simulink model "torque_control_model_3"  (R2017b)
settings: Solver=FixedStepAuto  StartTime=0.0  StopTime=.1  FixedStep=1e-6  RelTol=1e-3
InitFcn:
  | BLDC_motor_constants_2;
  | clc;
  | 
  | f=5000;           % Reference frequency
  | fs=4000;      % Switching frequency
  | m=1;           % Modulation index
  | 
  | Ts=10e-6;    % Sampling time of devices
values from neighbouring files (symbols this model uses):
  A = [-terminal_resistance/terminal_inductance, 0, 0 ... (first row only)    [BLDC_motor_constants_2.m]    (also in forward_dynamics.m = pinv(Z) * V; inverse_dynamics.m = -pinv(Z) * v)
  B = [2/(3 * terminal_inductance), 1/(3 * terminal_inductance), 0 ... (first row only)    [BLDC_motor_constants_2.m]    (also in forward_dynamics.m = pinv(Z)/gear_ratio)
  C = [1, 0, 0 ... (first row only)    [BLDC_motor_constants_2.m]
  kf = 0.001    [BLDC_motor_constants_2.m]
  pole_pairs = 8    [BLDC_motor_constants_2.m]
  rotor_inertia = 0.000181    [BLDC_motor_constants_2.m]
  speed_constant = 259    [BLDC_motor_constants_2.m]
  torque_constant = 36.9    [BLDC_motor_constants_2.m]
libraries: simulink x3
settings Model: Creator=Zach  LastModifiedBy=Zach

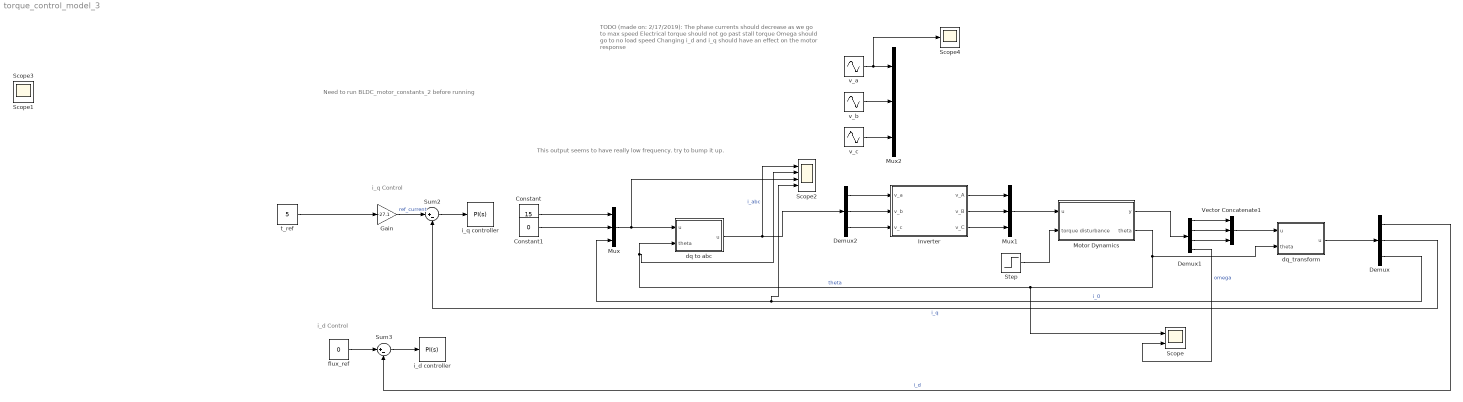
== system torque_control_model_3 ==
  note: TODO (made on: 2/17/2019):
      | The phase currents should decrease as we go to max speed
      | Electrical torque should not go past stall torque
      | Omega should go to no load speed
      | Changing i_d and i_q should have an effect on the motor response
  note: This output seems to have really low frequency. try to bump it up.
  note: i_d Control
  note: i_q Control
  note: Need to run BLDC_motor_constants_2 before running
  Constant : Constant  Value=15
  Constant1 : Constant  Value=0
  Demux : Demux  Outputs=3
  Demux1 : Demux
  Demux2 : Demux  Outputs=3
  Gain : Gain  Gain=-27.1
  Inverter : Subsystem
  Motor Dynamics : Subsystem
  Mux : Mux  Inputs=3
  Mux1 : Mux  Inputs=3
  Mux2 : Mux  Inputs=3
  Scope : Scope  NumInputPorts=2
  Scope2 : Scope  NumInputPorts=4
  Scope4 : Scope
  Step : Step  After=-.25  SampleTime=0
  Sum2 : Sum  Inputs=|+-
  Sum3 : Sum  Inputs=|+-
  Vector Concatenate1 : Concatenate  NumInputs=3
  dq to abc : MATLAB Function  TreatAsAtomicUnit=on
  dq_transform : MATLAB Function  TreatAsAtomicUnit=on
  flux_ref : Constant  Value=0
  i_d controller : simulink/Continuous/PID Controller  Controller=PI  TimeDomain=Continuous-time  SampleTime=-1  IntegratorMethod=Forward Euler  FilterMethod=Forward Euler  Form=Parallel  UseFilter=on  ControllerParametersSource=internal  P=20  I=1  D=0  N=100  InitialConditionSource=internal  InitialConditionForIntegrator=0  InitialConditionForFilter=0  ExternalReset=none  LimitOutput=off  UpperSaturationLimit=inf  LowerSaturationLimit=-inf  LinearizeAsGain=on  AntiWindupMode=none  Kb=1  TrackingMode=off  Kt=1  PParamMin=[]  PParamMax=[]  IParamMin=[]  IParamMax=[]  DParamMin=[]  DParamMax=[]  NParamMin=[]  NParamMax=[]  KbParamMin=[]  KbParamMax=[]  KtParamMin=[]  KtParamMax=[]  POutMin=[]  POutMax=[]  IOutMin=[]  IOutMax=[]  DOutMin=[]  DOutMax=[]  NOutMin=[]  NOutMax=[]  KbOutMin=[]  KbOutMax=[]  KtOutMin=[]  KtOutMax=[]  IntegratorOutMin=[]  IntegratorOutMax=[]  FilterOutMin=[]  FilterOutMax=[]  SumOutMin=[]  SumOutMax=[]  SumI1OutMin=[]  SumI1OutMax=[]  SumI2OutMin=[]  SumI2OutMax=[]  SumI3OutMin=[]  SumI3OutMax=[]  SumDOutMin=[]  SumDOutMax=[]  SaturationOutMin=[]  SaturationOutMax=[]  IntegratorContinuousStateAttributes=''  IntegratorStateMustResolveToSignalObject=off  IntegratorRTWStateStorageClass=Auto  FilterContinuousStateAttributes=''  FilterStateMustResolveToSignalObject=off  FilterRTWStateStorageClass=Auto  DifferentiatorICPrevScaledInput=0  DifferentiatorOutMin=[]  DifferentiatorOutMax=[]  InitialConditionSetting=State (most efficient)  FilterDiffOutCoefMin=[]  FilterDiffOutCoefMax=[]  SumDenOutMin=[]  SumDenOutMax=[]  SumNumOutMin=[]  SumNumOutMax=[]  ReciprocalOutMin=[]  ReciprocalOutMax=[]  DivideOutMin=[]  DivideOutMax=[]  TunerSelectOption=Transfer Function Based (PID Tuner App)
  i_q controller : simulink/Continuous/PID Controller  Controller=PI  TimeDomain=Continuous-time  SampleTime=-1  IntegratorMethod=Forward Euler  FilterMethod=Forward Euler  Form=Parallel  UseFilter=on  ControllerParametersSource=internal  P=1  I=1  D=0  N=100  InitialConditionSource=internal  InitialConditionForIntegrator=0  InitialConditionForFilter=0  ExternalReset=none  LimitOutput=off  UpperSaturationLimit=inf  LowerSaturationLimit=-inf  LinearizeAsGain=on  AntiWindupMode=none  Kb=1  TrackingMode=off  Kt=1  PParamMin=[]  PParamMax=[]  IParamMin=[]  IParamMax=[]  DParamMin=[]  DParamMax=[]  NParamMin=[]  NParamMax=[]  KbParamMin=[]  KbParamMax=[]  KtParamMin=[]  KtParamMax=[]  POutMin=[]  POutMax=[]  IOutMin=[]  IOutMax=[]  DOutMin=[]  DOutMax=[]  NOutMin=[]  NOutMax=[]  KbOutMin=[]  KbOutMax=[]  KtOutMin=[]  KtOutMax=[]  IntegratorOutMin=[]  IntegratorOutMax=[]  FilterOutMin=[]  FilterOutMax=[]  SumOutMin=[]  SumOutMax=[]  SumI1OutMin=[]  SumI1OutMax=[]  SumI2OutMin=[]  SumI2OutMax=[]  SumI3OutMin=[]  SumI3OutMax=[]  SumDOutMin=[]  SumDOutMax=[]  SaturationOutMin=[]  SaturationOutMax=[]  IntegratorContinuousStateAttributes=''  IntegratorStateMustResolveToSignalObject=off  IntegratorRTWStateStorageClass=Auto  FilterContinuousStateAttributes=''  FilterStateMustResolveToSignalObject=off  FilterRTWStateStorageClass=Auto  DifferentiatorICPrevScaledInput=0  DifferentiatorOutMin=[]  DifferentiatorOutMax=[]  InitialConditionSetting=State (most efficient)  FilterDiffOutCoefMin=[]  FilterDiffOutCoefMax=[]  SumDenOutMin=[]  SumDenOutMax=[]  SumNumOutMin=[]  SumNumOutMax=[]  ReciprocalOutMin=[]  ReciprocalOutMax=[]  DivideOutMin=[]  DivideOutMax=[]  TunerSelectOption=Transfer Function Based (PID Tuner App)
  t_ref : Constant  Value=5
  v_a : Sin  Frequency=pi*2*f  Phase=pi/2  SampleTime=0
  v_b : Sin  Frequency=f*2*pi  Phase=pi/2 -2*pi/3  SampleTime=0
  v_c : Sin  Frequency=12  Phase=pi/2+2*pi/3  SampleTime=0
  Scope1 : Scope
  Scope3 : Scope
  wires:
  Gain/1 -> Sum2/1  "ref_current"
  Sum2/1 -> i_q controller/1
  Demux/2 -> Sum2/2  "i_q"
  flux_ref/1 -> Sum3/1
  Sum3/1 -> i_d controller/1
  Demux/1 -> Sum3/2  "i_d"
  Demux/3 -> Scope2/4, Mux/3  "i_0"
  Step/1 -> Motor Dynamics/2(torque disturbance)
  Motor Dynamics/1(y) -> Demux1/1
  Demux1/2 -> Vector Concatenate1/2
  Demux1/1 -> Vector Concatenate1/1
  Demux1/3 -> Vector Concatenate1/3
  Motor Dynamics/2(theta) -> dq_transform/2(theta), Scope2/2, dq to abc/2(theta), Scope/1  "theta"
  Vector Concatenate1/1 -> dq_transform/1("u ")
  dq_transform/1(u) -> Demux/1
  Demux1/4 -> Scope/2  "omega"
  Constant/1 -> Mux/1
  Constant1/1 -> Mux/2
  t_ref/1 -> Gain/1
  Mux/1 -> Scope2/3, dq to abc/1("u ")
  Demux2/1 -> Inverter/1(v_a)
  Demux2/2 -> Inverter/2(v_b)
  Demux2/3 -> Inverter/3(v_c)
  Inverter/2(v_B) -> Mux1/2
  Inverter/1(v_A) -> Mux1/1
  Inverter/3(v_C) -> Mux1/3
  Mux1/1 -> Motor Dynamics/1(u)
  v_b/1 -> Mux2/2
  v_a/1 -> Scope4/1, Mux2/1
  v_c/1 -> Mux2/3
  dq to abc/1(u) -> Demux2/1, Scope2/1  "i_abc"

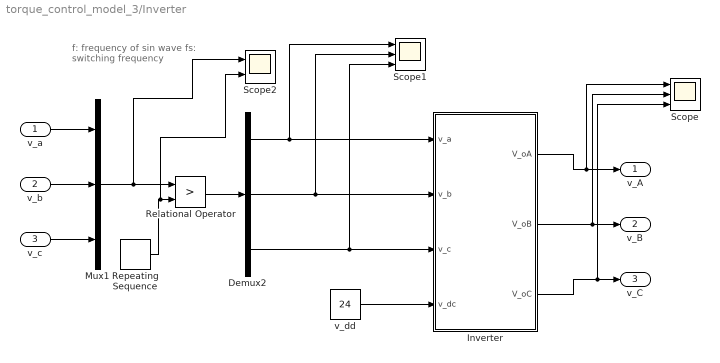
== system torque_control_model_3/Inverter ==
  note: f: frequency of sin wave
      | fs: switching frequency
  v_a : Inport
  v_b : Inport  Port=2
  v_c : Inport  Port=3
  Demux2 : Demux  Outputs=3
  Inverter : Subsystem
  Mux1 : Mux  Inputs=3
  Relational Operator : RelationalOperator  Operator=>  OutDataTypeStr=boolean  RndMeth=Simplest
  Repeating Sequence : simulink/Sources/Repeating Sequence  rep_seq_t=[0 0.25/fs 0.5/fs 0.75/fs 1/fs]  rep_seq_y=[1 0 -1 0 1]
  Scope : Scope  NumInputPorts=3
  Scope1 : Scope  NumInputPorts=3
  Scope2 : Scope  NumInputPorts=2
  v_dd : Constant  Value=24
  v_A : Outport
  v_B : Outport  Port=2
  v_C : Outport  Port=3
  wires:
  Relational Operator/1 -> Demux2/1
  Inverter/1(V_oA) -> Scope/1, v_A/1
  v_c/1 -> Mux1/3
  v_a/1 -> Mux1/1
  Demux2/3 -> Scope1/3, Inverter/3(v_c)
  Repeating Sequence/1 -> Scope2/2, Relational Operator/2
  v_b/1 -> Mux1/2
  Inverter/3(V_oC) -> Scope/3, v_C/1
  Demux2/1 -> Scope1/1, Inverter/1(v_a)
  Mux1/1 -> Scope2/1, Relational Operator/1
  v_dd/1 -> Inverter/4(v_dc)
  Demux2/2 -> Scope1/2, Inverter/2(v_b)
  Inverter/2(V_oB) -> Scope/2, v_B/1

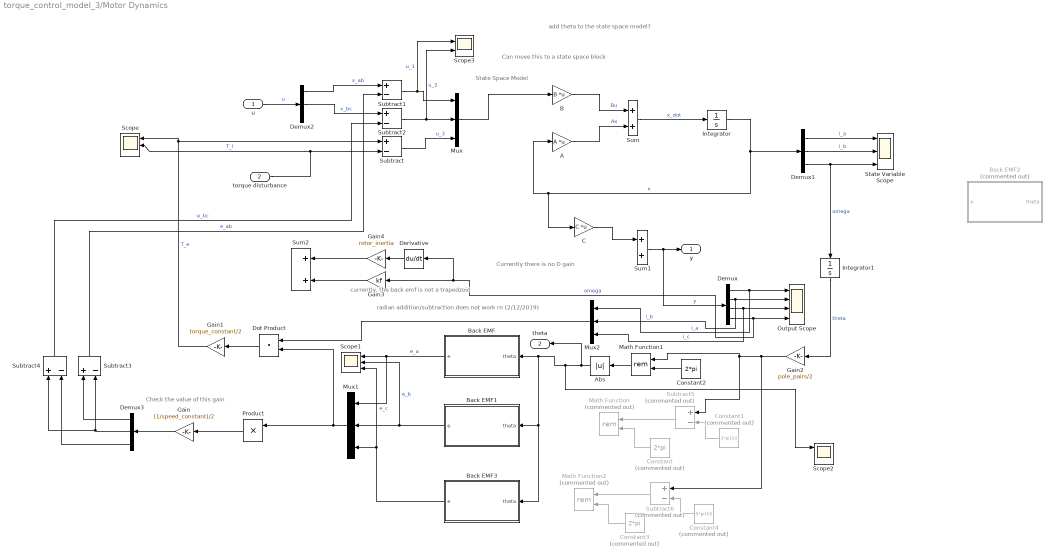
== system torque_control_model_3/Motor Dynamics ==
  note: radian addition/subtraction does not work rn (2/12/2019)
  note: add theta to the state space model?
  note: Check the value of this gain
  note: Can move this to a state space block
  note: currently, the back emf is not a trapedzoid
  note: Currently there is no D gain
  note: State Space Model
  u : Inport
  torque disturbance : Inport  Port=2
  A : Gain  Gain=A  Multiplication=Matrix(K*u)
  Abs : Abs
  B : Gain  Gain=B  Multiplication=Matrix(K*u)
  Back EMF : Subsystem
  Back EMF1 : Subsystem
  Back EMF2 : Subsystem  Commented=on
  Back EMF3 : Subsystem
  C : Gain  Gain=C  Multiplication=Matrix(K*u)
  Constant : Constant  Commented=on  Value=2*pi
  Constant1 : Constant  Commented=on  Value=2*pi()/3
  Constant2 : Constant  Value=2*pi
  Constant3 : Constant  Commented=on  Value=2*pi
  Constant4 : Constant  Commented=on  Value=5*pi()/3
  Demux : Demux
  Demux1 : Demux  Outputs=3
  Demux2 : Demux  Outputs=3
  Demux3 : Demux  Outputs=3
  Derivative : Derivative
  Dot Product : DotProduct  InputSameDT=on  OutDataTypeStr=Inherit: Inherit via internal rule
  Gain : Gain  Gain=(1/speed_constant)/2
  Gain1 : Gain  Gain=torque_constant/2
  Gain2 : Gain  Gain=pole_pairs/2
  Gain3 : Gain  Gain=kf
  Gain4 : Gain  Gain=rotor_inertia
  Integrator : Integrator
  Integrator1 : Integrator
  Math Function : Math  Commented=on  Operator=rem  SaturateOnIntegerOverflow=on
  Math Function1 : Math  Operator=rem  SaturateOnIntegerOverflow=on
  Math Function2 : Math  Commented=on  Operator=rem  SaturateOnIntegerOverflow=on
  Mux : Mux  Inputs=3
  Mux1 : Mux  Inputs=3
  Mux2 : Mux  Inputs=3
  Output Scope : Scope  NumInputPorts=4
  Product : Product
  Scope : Scope  NumInputPorts=3
  Scope1 : Scope  NumInputPorts=3
  Scope2 : Scope  NumInputPorts=3
  Scope3 : Scope  NumInputPorts=2
  State Variable Scope : Scope  NumInputPorts=3
  Subtract{,1..4} (5 alike) : Sum  Inputs=+-
  Subtract5 : Sum  Commented=on  Inputs=+-
  Subtract6 : Sum  Commented=on  Inputs=+-
  Sum : Sum
  Sum1 : Sum
  Sum2 : Sum
  y : Outport
  theta : Outport  Port=2
  wires:
  B/1 -> Sum/1  "Bu"
  A/1 -> Sum/2  "Ax"
  Sum/1 -> Integrator/1  "x_dot"
  Integrator/1 -> Demux1/1, C/1, A/1  "x"
  C/1 -> Sum1/1
  Sum1/1 -> Demux/1, y/1  "y"
  Demux/1 -> Mux2/1, Output Scope/1  "i_a"
  Demux/2 -> Mux2/2, Output Scope/2  "i_b"
  Demux/3 -> Mux2/3, Output Scope/3  "i_c"
  Demux/4 -> Derivative/1, Gain3/1, Output Scope/4  "omega"
  Demux1/1 -> State Variable Scope/1  "i_a"
  Demux1/2 -> State Variable Scope/2  "i_b"
  Demux1/3 -> State Variable Scope/3, Integrator1/1  "omega"
  Mux/1 -> B/1
  u/1 -> Demux2/1  "u"
  torque disturbance/1 -> Scope/2, Subtract/2  "T_l"
  Demux2/1 -> Subtract1/1  "v_ab"
  Demux2/2 -> Subtract2/1  "v_bc"
  Subtract2/1 -> Scope3/2, Mux/2  "u_2"
  Subtract1/1 -> Scope3/1, Mux/1  "u_1"
  Subtract/1 -> Mux/3  "u_3"
  Subtract3/1 -> Subtract1/2  "e_ab"
  Subtract4/1 -> Subtract2/2  "e_bc"
  Mux1/1 -> Dot Product/2, Product/1
  Product/1 -> Gain/1
  Gain/1 -> Demux3/1
  Demux3/1 -> Subtract3/1
  Demux3/2 -> Subtract4/1, Subtract3/2
  Demux3/3 -> Subtract4/2
  Mux2/1 -> Dot Product/1
  Dot Product/1 -> Gain1/1
  Gain1/1 -> Scope/1, Subtract/1  "T_e"
  Integrator1/1 -> Gain2/1  "theta"
  Constant/1 -> Math Function/2
  Constant1/1 -> Subtract5/2
  Subtract5/1 -> Math Function/1
  Constant2/1 -> Math Function1/2
  Constant4/1 -> Subtract6/2
  Constant3/1 -> Math Function2/2
  Subtract6/1 -> Math Function2/1
  Gain2/1 -> Subtract6/1, Subtract5/1, Math Function1/1
  Back EMF/1(e) -> Mux1/1, Scope1/1  "e_a"
  Back EMF1/1(e) -> Scope1/2, Mux1/2  "e_b"
  Back EMF3/1(e) -> Scope1/3, Mux1/3  "e_c"
  Derivative/1 -> Gain4/1
  Gain3/1 -> Sum2/2
  Gain4/1 -> Sum2/1
  Math Function1/1 -> Abs/1
  Abs/1 -> theta/1, Scope2/1, Back EMF3/1(theta), Back EMF1/1(theta), Back EMF/1(theta)

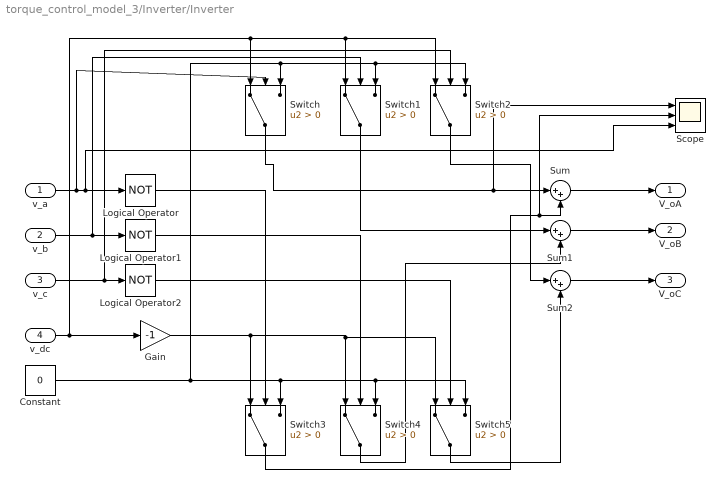
== system torque_control_model_3/Inverter/Inverter ==
  v_a : Inport
  v_b : Inport  Port=2
  v_c : Inport  Port=3
  v_dc : Inport  Port=4
  Constant : Constant  Value=0
  Gain : Gain  Gain=-1
  Logical Operator : Logic  Operator=NOT  AllPortsSameDT=off  OutDataTypeStr=boolean
  Logical Operator1 : Logic  Operator=NOT  AllPortsSameDT=off  OutDataTypeStr=boolean
  Logical Operator2 : Logic  Operator=NOT  AllPortsSameDT=off  OutDataTypeStr=boolean
  Scope : Scope  NumInputPorts=3
  Sum : Sum  Inputs=|++
  Sum1 : Sum  Inputs=|++
  Sum2 : Sum  Inputs=|++
  Switch{,1..5} (6 alike) : Switch  Criteria=u2 > Threshold
  V_oA : Outport
  V_oB : Outport  Port=2
  V_oC : Outport  Port=3
  wires:
  v_a/1 -> Switch/2, Scope/3, Logical Operator/1
  v_b/1 -> Switch1/2, Logical Operator1/1
  v_c/1 -> Switch2/2, Logical Operator2/1
  Logical Operator/1 -> Switch3/2
  Logical Operator1/1 -> Switch4/2
  Logical Operator2/1 -> Switch5/2
  v_dc/1 -> Switch2/1, Switch1/1, Switch/1, Gain/1
  Gain/1 -> Switch5/1, Switch4/1, Switch3/1
  Constant/1 -> Switch2/3, Switch1/3, Switch/3, Switch5/3, Switch4/3, Switch3/3
  Sum/1 -> V_oA/1
  Sum1/1 -> V_oB/1
  Sum2/1 -> V_oC/1
  Switch/1 -> Sum/1, Scope/1
  Switch3/1 -> Scope/2, Sum/2
  Switch1/1 -> Sum1/1
  Switch4/1 -> Sum1/2
  Switch2/1 -> Sum2/1
  Switch5/1 -> Sum2/2

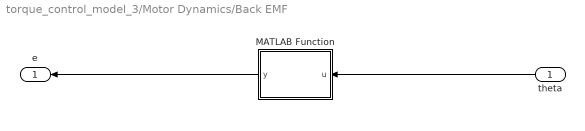
== system torque_control_model_3/Motor Dynamics/Back EMF ==
  theta : Inport
  MATLAB Function : MATLAB Function  TreatAsAtomicUnit=on
  e : Outport
  wires:
  theta/1 -> MATLAB Function/1(u)
  MATLAB Function/1(y) -> e/1

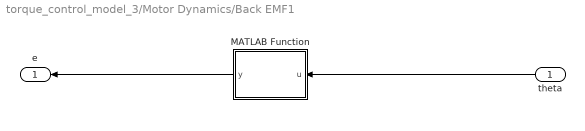
== system torque_control_model_3/Motor Dynamics/Back EMF1 ==
  theta : Inport
  MATLAB Function : MATLAB Function  TreatAsAtomicUnit=on
  e : Outport
  wires:
  MATLAB Function/1(y) -> e/1
  theta/1 -> MATLAB Function/1(u)

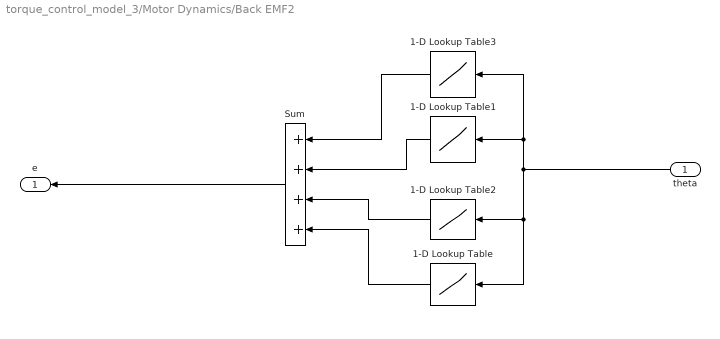
== system torque_control_model_3/Motor Dynamics/Back EMF2 ==
  theta : Inport
  1-D Lookup Table : Lookup_n-D  NumberOfTableDimensions=1  BreakpointsForDimension1=[0, 0.000001 ,2.08, 2.09]  Table=[0, 1,1, 0]  ExtrapMethod=Clip  UseLastTableValue=on  InternalRulePriority=Speed  RndMeth=Simplest  InputSameDT=on
  1-D Lookup Table1 : Lookup_n-D  NumberOfTableDimensions=1  BreakpointsForDimension1=[3.14158, 3.1416, 5.2, 5.2333 ]  Table=[0, -1, -1, 0]  ExtrapMethod=Clip  InternalRulePriority=Speed  RndMeth=Simplest  InputSameDT=on
  1-D Lookup Table2 : Lookup_n-D  NumberOfTableDimensions=1  BreakpointsForDimension1=[2.08, 2.0943951023931953,3.14158, 3.14159]  Table=[0, 1,-0.909859317102744, 0]  ExtrapMethod=Clip  InternalRulePriority=Speed  RndMeth=Simplest  InputSameDT=on
  1-D Lookup Table3 : Lookup_n-D  NumberOfTableDimensions=1  BreakpointsForDimension1=[5.2332, 5.234, 6.27, 6.28]  Table=[0, -1,1, 0]  ExtrapMethod=Clip  InternalRulePriority=Speed  RndMeth=Simplest  InputSameDT=on
  Sum : Sum  Inputs=4
  e : Outport
  wires:
  Sum/1 -> e/1
  theta/1 -> 1-D Lookup Table1/1, 1-D Lookup Table3/1, 1-D Lookup Table2/1, 1-D Lookup Table/1
  1-D Lookup Table1/1 -> Sum/2
  1-D Lookup Table/1 -> Sum/4
  1-D Lookup Table2/1 -> Sum/3
  1-D Lookup Table3/1 -> Sum/1

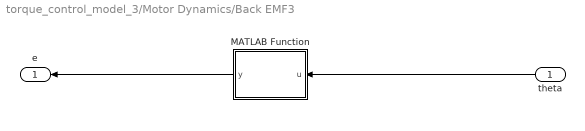
== system torque_control_model_3/Motor Dynamics/Back EMF3 ==
  theta : Inport
  MATLAB Function : MATLAB Function  TreatAsAtomicUnit=on
  e : Outport
  wires:
  MATLAB Function/1(y) -> e/1
  theta/1 -> MATLAB Function/1(u)

== matlab function torque_control_model_3/dq to abc ==
  data: u input; u output; theta input
function u = fcn(u, theta)
pole_pairs = 8; %Figure out how to pull this from the workspace
transform = sqrt(2/3) * ...
     [cos(theta * pole_pairs), cos((theta * pole_pairs) - 2*pi()/3), cos(((theta * pole_pairs) + 2*pi()/3));
     -sin(theta * pole_pairs), -sin(((theta * pole_pairs) - 2*pi()/3)), -sin(((theta * pole_pairs) + 2*pi()/3));
     1/sqrt(2), 1/sqrt(2), 1/sqrt(2)]';
u = transform * u;

== matlab function torque_control_model_3/dq_transform ==
  data: u input; u output; theta input
function u = fcn(u, theta)
pole_pairs = 8; %Figure out how to pull this from the workspace
transform = sqrt(2/3) * ...
     [cos(theta * pole_pairs), cos((theta * pole_pairs) - 2*pi()/3), cos((theta * pole_pairs) + 2*pi()/3);
     -sin(theta * pole_pairs), -sin((theta * pole_pairs) - 2*pi()/3), -sin((theta * pole_pairs) + 2*pi()/3);
     1/sqrt(2), 1/sqrt(2), 1/sqrt(2)];
u = transform * u;

== matlab function torque_control_model_3/Motor Dynamics/Back EMF/MATLAB Function ==
  data: u input; y output
function y = fcn(u)
y = 0;
%u = abs(rem(u, 2*pi()));
if (0 <= u && u < 2*pi()/3)
    y = 1;
elseif (2*pi()/3 <= u && u < pi())
    y = 1 - (6/pi())*(u - (2*pi()/3));
elseif (pi() <= u && u < (5*pi()/3))
    y = -1;
else
    y = -1 + (6/pi())*(u - (5*pi()/3));
end

== matlab function torque_control_model_3/Motor Dynamics/Back EMF1/MATLAB Function ==
  data: u input; y output
function y = fcn(u)
y = 0;
% u = abs(rem(u, 2*pi()));
% u = u - (2*pi()/3);

% if u < 0
%      u = 2*pi() + u;
% end

if (0 <= u && u < pi()/3)
    y = -1;
elseif (pi()/3 <= u && u < 2*pi()/3)
    y = -1 + (6/pi())*(u - (pi()/3));
elseif (2*pi()/3 <= u && u < (4*pi()/3))
    y = 1;
elseif ((4*pi()/3) <= u && u < 5*pi()/3)
    y = 1 - ((6/pi()) * (u - (4*pi()/3)));
elseif (5*pi()/3 <= u && u < 2*pi())
    y = -1;
end

== matlab function torque_control_model_3/Motor Dynamics/Back EMF3/MATLAB Function ==
  data: u input; y output
function y = fcn(u)
y = 0;
% u = u - (4*pi()/3);
% u = abs(rem(u, 2*pi()));

% if u < 0
%      u = 2*pi() + u;
% end

if (0 <= u && u < pi()/3)
    y = 1 - (6/pi())*(u);
elseif (pi()/3 <= u && u < pi())
    y = -1;
elseif (pi() <= u && u < (4*pi()/3))
    y = -1 + (6/pi())*(u - pi());
elseif ((4*pi()/3) <= u < 2*pi())
    y = 1;
end
